simulink model "chap1_3"  (Simulink 3.00)
settings: Solver=ode45  StartTime=0.0  StopTime=10.0  RelTol=1e-3
libraries: simulink3 x1

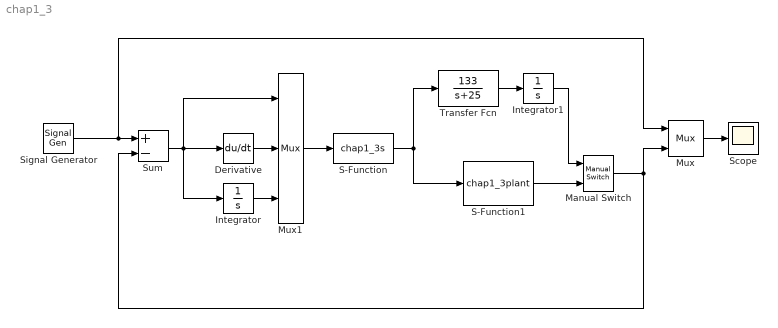
== system chap1_3 ==
  Derivative : Derivative
  Integrator : Integrator  ExternalReset=none  InitialConditionSource=internal  InitialCondition=0  LimitOutput=off  UpperSaturationLimit=inf  LowerSaturationLimit=-inf  ShowSaturationPort=off  ShowStatePort=off  AbsoluteTolerance=auto
  Integrator1 : Integrator  ExternalReset=none  InitialConditionSource=internal  InitialCondition=0  LimitOutput=off  UpperSaturationLimit=inf  LowerSaturationLimit=-inf  ShowSaturationPort=off  ShowStatePort=off  AbsoluteTolerance=auto
  Manual Switch : simulink3/Nonlinear/Manual Switch  sw=0  action=0
  Mux : Mux  Inputs=2
      settings: DisplayOption=none
  Mux1 : Mux  Inputs=3
      settings: DisplayOption=none
  S-Function : S-Function  FunctionName=chap1_3s  PortCounts=[]  SFunctionModules=''
  S-Function1 : S-Function  FunctionName=chap1_3plant  PortCounts=[]  SFunctionModules=''
  Scope : Scope
      settings: TimeRange=8  YMin=-1.5  YMax=1.5  SaveToWorkspace=off  SaveName=ScopeData  MaxRows=50000
  Signal Generator : SignalGenerator  WaveForm=sine  Amplitude=1  Frequency=0.2  Units=Hertz
  Sum : Sum  Inputs=+-  SaturateOnIntegerOverflow=on
  Transfer Fcn : TransferFcn  Numerator=[133]  Denominator=[1 25]
  wires:
  Signal Generator/1 -> Sum/1, Mux/1
  Mux/1 -> Scope/1
  S-Function/1 -> Transfer Fcn/1, S-Function1/1
  S-Function1/1 -> Manual Switch/2
  Manual Switch/1 -> Mux/2, Sum/2
  Mux1/1 -> S-Function/1
  Derivative/1 -> Mux1/2
  Integrator/1 -> Mux1/3
  Sum/1 -> Mux1/1, Derivative/1, Integrator/1
  Transfer Fcn/1 -> Integrator1/1
  Integrator1/1 -> Manual Switch/1
